simulink model "evenOdd"  (R2021a)
settings: Solver=FixedStepDiscrete  StartTime=0.0  StopTime=10.0  RelTol=1e-3  EnableMultiTasking=on
libraries: simulink x1, embmathops x1
settings Model: Creator=iT-User  LastModifiedBy=iT-User
settings DataIOCC: ReturnWorkspaceOutputs=off
settings OptimizationCC: DefaultParameterBehavior=Inlined  InlineInvariantSignals=on  EnableMemcpy=off  LifeSpan=1  EfficientTunableParamExpr=on
settings DebuggingCC: UnderspecifiedInitializationDetection=Classic  MergeDetectMultiDrivingBlocksExec=none  SFMachineParentedDataDiag=warning  ArithmeticOperatorsInVariantConditions=warning
settings ModelReferenceCC: PropagateSignalLabelsOutOfModel=off
settings SFSimCC: MATLABDynamicMemAlloc=off  CustomCodeUndefinedFunction=UseInterfaceOnly
settings RTWCC: SystemTargetFile=ert.tlc  GenCodeOnly=on  TemplateMakefile=ert_default_tmf  GenerateReport=on  IncludeHyperlinkInReport=on  LaunchReport=on  GenerateTraceInfo=on  GenerateTraceReport=on  GenerateTraceReportSl=on  GenerateTraceReportSf=on  GenerateTraceReportEml=on
settings CodeAppCC: ForceParamTrailComments=on  IgnoreCustomStorageClasses=off  OperatorAnnotations=on  SimulinkDataObjDesc=on  SFDataObjDesc=on  MATLABFcnDesc=on  InsertBlockDesc=on  StateflowObjectComments=on  MATLABSourceComments=on
settings ERTTargetCC: MultiwordLength=2048  GenerateSampleERTMain=on  InlinedParameterPlacement=NonHierarchical  ERTCustomFileTemplate=example_file_process.tlc

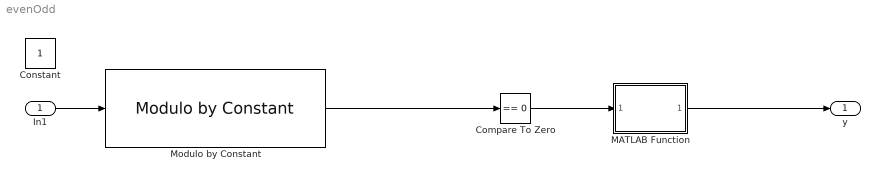
== system evenOdd ==
  In1 : Inport
  Compare To Zero : simulink/Logic and Bit Operations/Compare To Zero  relop===  OutDataTypeStr=uint8
  Constant : Constant
  MATLAB Function : MATLAB Function  TreatAsAtomicUnit=on
  Modulo by Constant : embmathops/Modulo by Constant  Denominator=2  SimulateUsing=Code generation
      settings: SourceProductBaseCode=SL
  y : Outport  OutDataTypeStr=string
  wires:
  Modulo by Constant/1 -> Compare To Zero/1
  In1/1 -> Modulo by Constant/1
  Compare To Zero/1 -> MATLAB Function/1(inputValue)
  MATLAB Function/1(outputValue) -> y/1

== matlab function evenOdd/MATLAB Function ==
  data: inputValue input; outputValue output
function outputValue = fcn(inputValue)

    if inputValue == 0
        outputValue = "odd"; % Use a numeric value to represent 'even'
    else
        outputValue = "even"; % Use a numeric value to represent 'odd'
    end
end
